simulink model "controller1"  (R2024a)
settings: Solver=VariableStepAuto  StartTime=0.0  StopTime=500  RelTol=1e-3
libraries: cstblocks x1
settings Model: Creator=stanleychiu  LastModifiedBy=stanleychiu

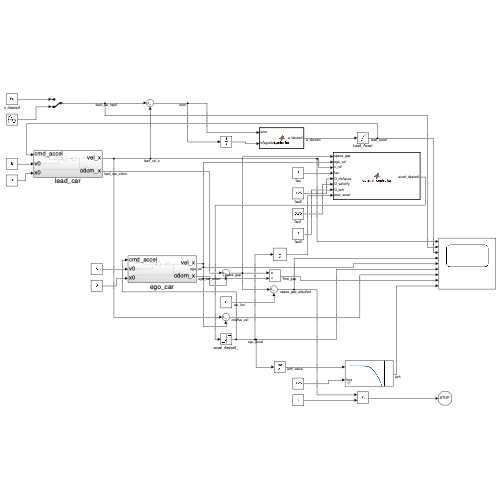
[thumbnail: Simulink's stored preview of the top-level diagram]
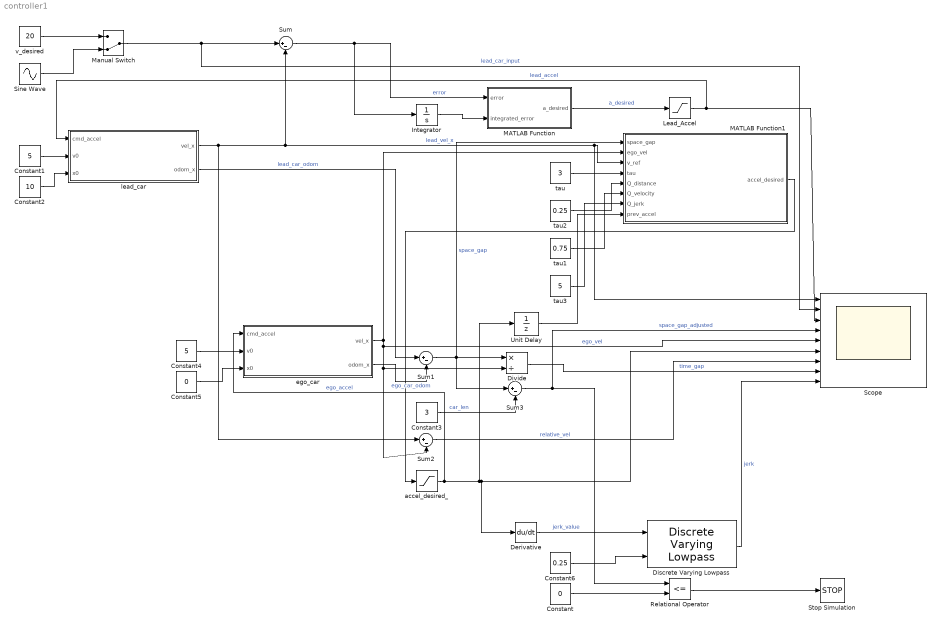
== system controller1 ==
  Constant : Constant  Value=0
  Constant1 : Constant  Value=5
  Constant2 : Constant  Value=10
  Constant3 : Constant  Value=3
  Constant4 : Constant  Value=5
  Constant5 : Constant  Value=0
  Constant6 : Constant  Value=0.25
  Derivative : Derivative
  Discrete Varying Lowpass : cstblocks/Linear Parameter Varying/Discrete Varying Lowpass  N=1  w0=0  Ts=0.1
  Divide : Product  Inputs=*/
  Integrator : Integrator
  Lead_Accel : Saturate  UpperLimit=1.5  LowerLimit=-3
  MATLAB Function : MATLAB Function  TreatAsAtomicUnit=on
  MATLAB Function1 : MATLAB Function  TreatAsAtomicUnit=on
  Manual Switch : ManualSwitch  CurrentSetting=0
  Relational Operator : RelationalOperator  Operator=<=  OutDataTypeStr=boolean  RndMeth=Simplest  InputSameDT=off
  Scope : Scope  NumInputPorts=9
  Sine Wave : Sin  Bias=20  SampleTime=0
  Stop Simulation : Stop
  Sum{,1..3} (4 alike) : Sum  Inputs=|+-
  Unit Delay : UnitDelay  SampleTime=-1  HasFrameUpgradeWarning=on
  accel_desired_ : Saturate  UpperLimit=20  LowerLimit=-20
  ego_car : Subsystem
  lead_car : Subsystem
  tau : Constant  Value=3
  tau1 : Constant  Value=0.75
  tau2 : Constant  Value=0.25
  tau3 : Constant  Value=5
  v_desired : Constant  Value=20
  wires:
  Relational Operator/1 -> Stop Simulation/1
  Discrete Varying Lowpass/1 -> Scope/9  "jerk"
  MATLAB Function1/1(accel_desired) -> accel_desired_/1
  Lead_Accel/1 -> Scope/3, lead_car/1(cmd_accel)  "lead_accel"
  Constant/1 -> Relational Operator/2
  Constant6/1 -> Discrete Varying Lowpass/2
  Derivative/1 -> Discrete Varying Lowpass/1  "jerk_value"
  Sum3/1 -> Relational Operator/1, Scope/4  "space_gap_adjusted"
  Divide/1 -> Scope/8  "time_gap"
  Unit Delay/1 -> MATLAB Function1/8(prev_accel)
  tau2/1 -> MATLAB Function1/5(Q_distance)
  Constant1/1 -> lead_car/2(v0)
  MATLAB Function/1(a_desired) -> Lead_Accel/1  "a_desired"
  Sum2/1 -> Scope/7  "relative_vel"
  Constant3/1 -> Sum3/2  "car_len"
  tau1/1 -> MATLAB Function1/6(Q_velocity)
  Sum1/1 -> Sum3/1, MATLAB Function1/1(space_gap), Divide/1  "space_gap"
  lead_car/2(odom_x) -> Sum1/1  "lead_car_odom"
  accel_desired_/1 -> Derivative/1, Scope/6, Unit Delay/1, ego_car/1(cmd_accel)  "ego_accel"
  lead_car/1(vel_x) -> Scope/1, MATLAB Function1/3(v_ref), Sum/2, Sum2/1  "lead_vel_x"
  Constant5/1 -> ego_car/3(x0)
  Constant4/1 -> ego_car/2(v0)
  Constant2/1 -> lead_car/3(x0)
  tau/1 -> MATLAB Function1/4(tau)
  ego_car/1(vel_x) -> Sum2/2, Divide/2, Scope/5, MATLAB Function1/2(ego_vel)  "ego_vel"
  Sine Wave/1 -> Manual Switch/2
  tau3/1 -> MATLAB Function1/7(Q_jerk)
  ego_car/2(odom_x) -> Sum1/2  "ego_car_odom"
  v_desired/1 -> Manual Switch/1
  Sum/1 -> Integrator/1, MATLAB Function/1(error)  "error"
  Integrator/1 -> MATLAB Function/2(integrated_error)
  Manual Switch/1 -> Sum/1, Scope/2  "lead_car_input"

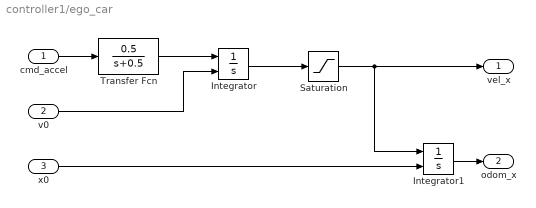
== system controller1/ego_car ==
  cmd_accel : Inport
  v0 : Inport  Port=2
  x0 : Inport  Port=3
  Integrator : Integrator  InitialConditionSource=external
  Integrator1 : Integrator  InitialConditionSource=external
  Saturation : Saturate  UpperLimit=80  LowerLimit=0
  Transfer Fcn : TransferFcn  Numerator=[0.5]  Denominator=[1 0.5]
  vel_x : Outport
  odom_x : Outport  Port=2
  wires:
  v0/1 -> Integrator/2
  cmd_accel/1 -> Transfer Fcn/1
  Transfer Fcn/1 -> Integrator/1
  Integrator1/1 -> odom_x/1
  Integrator/1 -> Saturation/1
  x0/1 -> Integrator1/2
  Saturation/1 -> vel_x/1, Integrator1/1

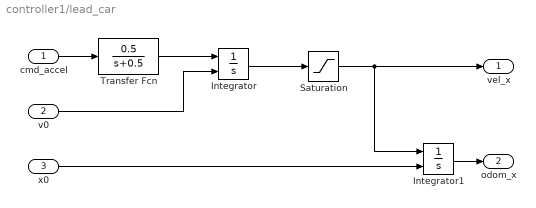
== system controller1/lead_car ==
  cmd_accel : Inport
  v0 : Inport  Port=2
  x0 : Inport  Port=3
  Integrator : Integrator  InitialConditionSource=external
  Integrator1 : Integrator  InitialConditionSource=external
  Saturation : Saturate  UpperLimit=80  LowerLimit=0
  Transfer Fcn : TransferFcn  Numerator=[0.5]  Denominator=[1 0.5]
  vel_x : Outport
  odom_x : Outport  Port=2
  wires:
  v0/1 -> Integrator/2
  cmd_accel/1 -> Transfer Fcn/1
  Transfer Fcn/1 -> Integrator/1
  Integrator1/1 -> odom_x/1
  Integrator/1 -> Saturation/1
  x0/1 -> Integrator1/2
  Saturation/1 -> vel_x/1, Integrator1/1

== matlab function controller1/MATLAB Function1 ==
  data: space_gap input; accel_desired output; ego_vel input; v_ref input; tau input; Q_distance input; Q_velocity input; Q_jerk input; prev_accel input
function accel_desired = optimal_controller(space_gap, ego_vel, v_ref, tau, Q_distance, Q_velocity, Q_jerk, prev_accel)
    % Inputs:
    % space_gap: Current gap between the ego vehicle and the lead vehicle
    % ego_vel: Current velocity of the ego vehicle
    % v_ref: Reference velocity (desired velocity or lead vehicle velocity)
    % tau: Time gap (constant time gap parameter)
    % Q_distance: Weight for space gap penalty
    % Q_velocity: Weight for velocity penalty
    % Q_jerk: Weight for jerk penalty
    % prev_accel: Previous acceleration (used to compute jerk)
    
    % Define the desired space gap based on the time gap
    desired_gap = ego_vel * tau;

    % Set bounds for acceleration (e.g., physical limits of the vehicle)
    accel_min = -3;  % Minimum allowed acceleration (e.g., maximum braking)
    accel_max = 1.5;   % Maximum allowed acceleration (e.g., maximum acceleration)
    
    % Define the cost function: we aim to minimize space gap, velocity deviations, and jerk
    cost_function = @(a) ...
        Q_distance * (space_gap - desired_gap)^2 + ...  % Space gap penalty
        Q_velocity * (ego_vel + a - v_ref)^2 + ...      % Velocity penalty
        Q_jerk * (a - prev_accel)^2;                   % Jerk penalty (rate of change of acceleration)
    
    % Optimization to minimize the cost function subject to acceleration limits
    options = optimoptions('fmincon', 'Algorithm', 'sqp', 'Display', 'off');
    accel_desired = fmincon(cost_function, prev_accel, [], [], [], [], accel_min, accel_max, [], options);
end

== matlab function controller1/MATLAB Function ==
  data: error input; a_desired output; integrated_error input
function a_desired = controller(error,integrated_error)

a_desired = 0.3*error + 0.01*integrated_error;
